simulink model "oUmControlador"  (R2018a)
settings: Solver=VariableStepAuto  StartTime=0.0  StopTime=10.0  RelTol=1e-3
settings Model: Creator=vittorfp  LastModifiedBy=dessa

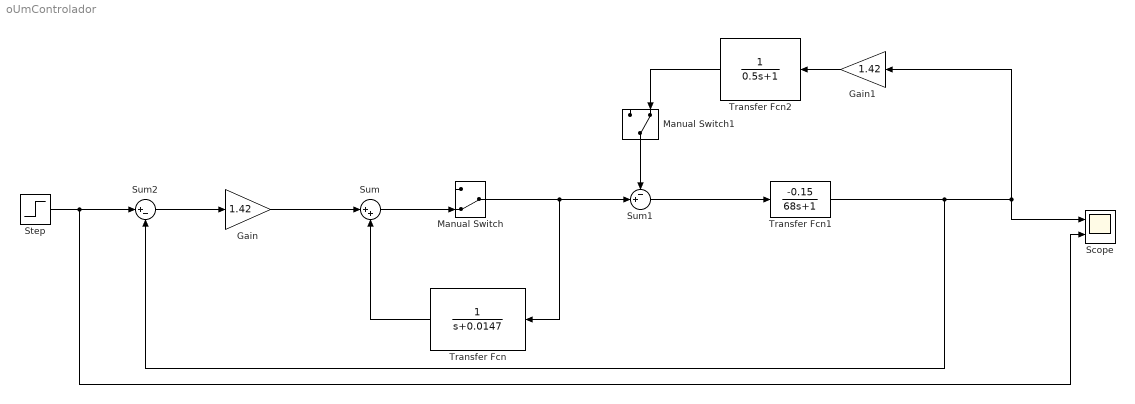
== system oUmControlador ==
  Gain : Gain  Gain=1.42
  Gain1 : Gain  Gain=1.42
  Manual Switch : ManualSwitch  CurrentSetting=0
  Manual Switch1 : ManualSwitch  CurrentSetting=0
  Scope : Scope  NumInputPorts=2
  Step : Step  After=20  SampleTime=0
  Sum : Sum  Inputs=|++
  Sum1 : Sum  Inputs=-+|
  Sum2 : Sum  Inputs=|+-
  Transfer Fcn : TransferFcn  Denominator=[1 0.0147]
  Transfer Fcn1 : TransferFcn  Numerator=[-0.15]  Denominator=[68 1]
  Transfer Fcn2 : TransferFcn  Denominator=[0.5 1]
  wires:
  Gain/1 -> Sum/1
  Sum/1 -> Manual Switch/2
  Manual Switch/1 -> Sum1/2, Transfer Fcn/1
  Transfer Fcn/1 -> Sum/2
  Sum1/1 -> Transfer Fcn1/1
  Gain1/1 -> Transfer Fcn2/1
  Transfer Fcn1/1 -> Sum2/2, Gain1/1, Scope/1
  Sum2/1 -> Gain/1
  Step/1 -> Scope/2, Sum2/1
  Manual Switch1/1 -> Sum1/1
  Transfer Fcn2/1 -> Manual Switch1/2
